simulink model "passiveBalancing"  (R2020b)
settings: Solver=ode23t  StartTime=0.0  StopTime=3600 * 15  MaxStep=.5  RelTol=1e-3  AbsTol=1e-3  EnableMultiTasking=on
PreLoadFcn:
  | passiveBalancing_ini;
model workspace (MAT data in the model file):
  Switch = 1
values from neighbouring files (symbols this model uses):
  I_cc = 4    [passiveBalancing_ini.m]
  I_gain = 10    [passiveBalancing_ini.m]
  P_gain = 100    [passiveBalancing_ini.m]
  R_bleed = 20    [passiveBalancing_ini.m]
  T_f = 600    [passiveBalancing_ini.m]
  V_top = 4.1    [passiveBalancing_ini.m]
libraries: fl_lib x15, nesl_utility x15, ee_lib x6, simulink x1, pid_lib x1
(part 1 of 2)
settings Model: PacingRate=100000  Creator=Amrathesh  LastModifiedBy=amrat
settings SolverCC: AutoScaleAbsTol=off  ZeroCrossAlgorithm=Adaptive
settings DataIOCC: LimitDataPoints=on  SaveOutput=off  SignalLogging=off  SaveTime=off  ReturnWorkspaceOutputs=off
settings OptimizationCC: DefaultParameterBehavior=Inlined  LifeSpan=2  EfficientTunableParamExpr=on
settings DebuggingCC: AlgebraicLoopMsg=error  AllowSymbolicDim=off  PregeneratedLibrarySubsystemCodeDiagnostic=none  SFUnexpectedBacktrackingDiag=warning  SFNoUnconditionalDefaultTransitionDiag=none  SFExecutionAtInitializationDiag=none  ArithmeticOperatorsInVariantConditions=warning
settings HardwareCC: ProdWordSize=32
settings ModelReferenceCC: PropagateSignalLabelsOutOfModel=off
settings SFSimCC: SimUseLocalCustomCode=off  MATLABDynamicMemAlloc=off  CustomCodeUndefinedFunction=UseInterfaceOnly
settings RTWCC: Description=Embedded Coder  SystemTargetFile=ert.tlc  TemplateMakefile=ert_default_tmf  GenerateReport=on  RTWUseLocalCustomCode=off  IncludeHyperlinkInReport=on  LaunchReport=on  GenerateTraceInfo=on  GenerateTraceReport=on  GenerateTraceReportSl=on  GenerateTraceReportSf=on  GenerateTraceReportEml=on
settings CodeAppCC: ForceParamTrailComments=on  IgnoreCustomStorageClasses=off  OperatorAnnotations=on  SimulinkDataObjDesc=on  SFDataObjDesc=on  MATLABFcnDesc=on  InsertBlockDesc=on  StateflowObjectComments=on  MATLABSourceComments=on
settings ERTTargetCC: MultiwordLength=2048  GenerateSampleERTMain=on  InlinedParameterPlacement=NonHierarchical  ERTCustomFileTemplate=example_file_process.tlc
settings ConfigComp: CovMetricSettings=dw  CovSaveCumulativeToWorkspaceVar=on  CovSaveSingleToWorkspaceVar=on  CovExternalEMLEnable=off
settings SimscapeCC: SimscapeNormalizeSystem=off  SimscapeLogType=all  SimscapeLogToSDI=on  SimscapeLogDataHistory=10000

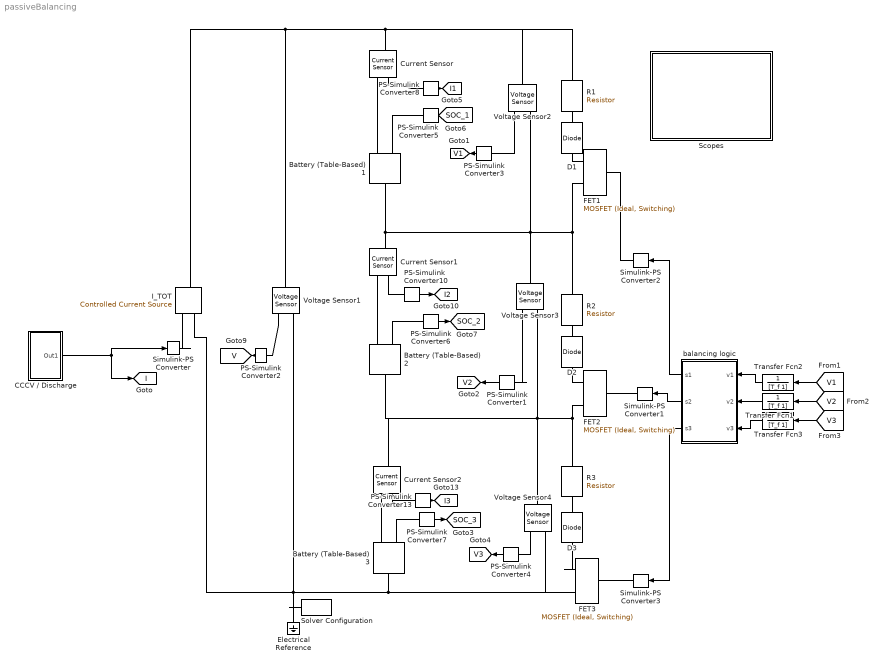
== system passiveBalancing ==
  Battery (Table-Based)1 : ee_lib/Sources/Battery (Table-Based)  Tag={'toolbox/physmod/elec/library/m/ee_lib_parts';'Sources/Battery__Table_Based_/Panasonic/UR18650A.xml'}  SOC_vec=[0.100000000000000;0.200000000000000;0.300000000000000;0.400000000000000;0.500000000000000;0.600000000000000;0.700000000000000;0.800000000000000;0.900000000000000;1]  T_dependence=ee.enum.temperature_dependence.yes  prm_dir=ee.enum.battery.prm_dir.noCurrentDirectionality  T_vec=[278.150000000000,293.150000000000,313.150000000000] K  V0_mat=[3.48407194875853,3.49373906253632,3.50592874552606;3.55418080716149,3.55259570558520,3.55508312112845;3.60440404431230,3.61410230902054,3.61515360383738;3.64321489304947,3.64896659680084,3.65685703896214;3.68502177847119,3.68864192779988,3.69639679484736;3.74422605890089,3.74398921633946,3.75105784288072;3.82967867350671,3.83940080415011,3.85325138336218;3.94315917033962,3.94854312702762,3.95608335309560;4.05943812577673,4.06094828281537,4.06565632904983;4.19049029477082,4.19030181290971,4.18799231154579] V  V0_vec=[2.81006584508995 3.22022478679487 3.35333985530666 3.4210479419583 3.43340289744142 3.44901435079157 3.46164239061189 3.47280320112771 3.47971224601289 3.48236456069527 3.48683507881654 3.49335561249342 3.49763390170867 3.50163709058121 3.50680001394047 3.51219805506247 3.51751682512439 3.52259342518673 3.52865552184197 3.53316807350089 3.53768062515982 3.54219317681874 3.54670572847766 3.55143972547218 3.55647692760588 3.56168247719111 3.56694531744751 3.57220815770393 3.57747099796033 3.58273383821674 3.5875530992875 3.59176313859395 3.59524803726717 3.59891401218516 3.60257998710315 3.60624596202113 3.61006223866338 3.61403025053352 3.61799826240367 3.62196627427381 3.62727855718798 3.6319884367608 3.63698876786423 3.64203407138805 3.64707937491187 3.65212467843569 3.65716998195951 3.66221528548332 3.66729939294707 3.67295160796092 3.67881814753232 3.68468468710373 3.69055122667513 3.69641776624653 3.70184846811763 3.70677938326847 3.71171029841932 3.71666876915231 3.72316392974375 3.7304733189824 3.73778270822105 3.745036871918 3.75209516011368 3.75915344830935 3.76621173650503 3.77398066542743 3.78333553443086 3.7926451126744 3.80054605529622 3.80844699791802 3.81634794053984 3.82429836269964 3.83446027504896 3.84531418436014 3.85639886265616 3.86778116509702 3.87916346753789 3.89054576997875 3.90044812182432 3.91099190865954 3.92153569549475 3.93213383878664 3.94271770825583 3.95339662764836 3.96407554704089 3.97475446643342 3.9856014296663 3.99763743545176 4.00976952670118 4.02190161795059 4.03372971668446 4.04698942952056 4.06070820502709 4.07426940349866 4.08362358507044 4.0946516607131 4.10632109738002 4.11746763572909 4.13600949794925 4.11358192572688] V  R0_mat=[0.0164025520353838,0.00991391593917779,0.00933168437168862;0.0119600956597842,0.00875043635238341,0.00956154423893035;0.0119853068610826,0.00832297953681552,0.00854455182155223;0.0111330643324705,0.00872061850253288,0.00956139374993682;0.0118222895857250,0.00795909444960185,0.00880754790179610;0.0116748342939053,0.00856548056926203,0.00938193010301517;0.0112768580015193,0.00843330788647423,0.00996649091964517;0.0118933795996695,0.00850334186162495,0.00960019659194077;0.0120321348242062,0.00846602435735512,0.00963753251603531;0.0124098156482057,0.00846539753229566,0.00929821710866923] Ohm  R0_vec=[0.056515741669998 0.0979844967251839 0.0915569898783186 0.0798231515434287 0.0702524951827934 0.0654000373090211 0.063093856936673 0.0616308263389111 0.0599710561216984 0.057768198464152 0.0561995978201733 0.0555761442485201 0.0546523884163435 0.0536806499662514 0.0531134700580429 0.0526283079740431 0.0521431458900432 0.0516579838060416 0.0515369348195236 0.0512705771965729 0.0510042195736231 0.0507378619506724 0.0504715043277217 0.0502823950776516 0.0502561644624615 0.0502595683975375 0.0502729648915397 0.0502863613855435 0.0502997578795457 0.0503131543735487 0.0503265508675508 0.0502574673059781 0.0501120429454529 0.0500297847168234 0.0499475264881939 0.0498652682595635 0.0497830100309331 0.0497007518023036 0.0496184935736741 0.0495362353450446 0.0496803807796349 0.0495816760338741 0.0494829712881124 0.0493842665423516 0.0492855617965899 0.04918685705083 0.0490881523050684 0.0489894475593067 0.0488907428135468 0.0488792431935741 0.0489051257638717 0.0489310083341703 0.0489568909044689 0.0489827734747674 0.048856619637978 0.0485561215964543 0.0482556235549287 0.0479551255134041 0.0478887983616394 0.047964487834391 0.0480401773071417 0.0480966020560407 0.0480846981417065 0.0480727942273722 0.048060890313038 0.0481036878566563 0.04837530229414 0.0486311176293377 0.0483955484453293 0.0481599792613174 0.0479244100773082 0.0476974710452733 0.0478971482990236 0.0483382198417974 0.0487792913845713 0.0492203629273451 0.0496614344701189 0.0501025060128928 0.0499772096727922 0.0499177661458976 0.049858322619003 0.0497988790921067 0.0497828516280938 0.0498086176006431 0.0498343835731925 0.0498601495457418 0.0499152254904454 0.0500578808408836 0.0502005361913236 0.0503431915417627 0.0503798029914302 0.0505673178409918 0.0508126169361116 0.0509278793074452 0.049575577643969 0.0485152342486694 0.0475667561482966 0.0457576853133315 0.0447350638775861 0.0121745905370672] Ohm  R0_dis_mat=[0.03 0.015 0.002;0.04 0.017 0.008;0.039 0.012 0.006;0.027 0.013 0.021] % Parameter not set Ohm  R0_dis_vec=[0.015 0.017 0.012 0.013] % Parameter not set Ohm  R0_ch_mat=[0.03 0.015 0.002;0.04 0.017 0.008;0.039 0.012 0.006;0.027 0.013 0.021] % Parameter not set Ohm  R0_ch_vec=[0.015 0.017 0.012 0.013] % Parameter not set Ohm  AH_vec=[1.82394991873531 2.0165 2.32772554803559] hr*A  AH=2.05260817612401 hr*A  prm_leak=ee.enum.battery.prm_leak.disabled  Rleak_vec=[8000 7000 6000] % Parameter not set Ohm  Rleak=7000 % Parameter not set Ohm  extrapolation_option=ee.enum.extrapolation.linear  prm_dyn=ee.enum.battery.prm_dyn.rc3  R1_mat=[0.00470517937000299,0.000293638394729167,0.000948546678306262;0.00290275050725254,0.000906415294998030,0.000287127543931831;0.00173884757466172,0.00126508138885500,0.00118355047696410;0.00166867739185738,0.000314621823867429,0.000269194023197089;0.000922417169458259,0.00115254740207724,0.000615957962246520;0.00120601315196432,0.000484496431848577,0.000263719105084760;0.00134107014418335,0.000722662778209487,4.84440937939109e-05;0.00102728323615524,0.000788593565891369,0.000287482375984320;0.00107112644740310,0.000808964645885711,0.000207425991333054;0.00109762911159868,0.000794632163172680,0.000106864004690497] Ohm  R1_vec=[0.076 0.022 0.007 0.043] % Parameter not set Ohm  tau1_mat=[13.5871605581300,9.71544043458337,4.31542721208131;12.5481735435305,12.1200192117783,22.7640233955017;7.48337010487386,12.0370710856561,8.29042934523224;9.44542449719648,10.9054745144726,9.51113592097300;9.24780665009956,9.25131458132309,4.68694878468948;13.0193706450093,13.4646058128269,7.73065506391290;11.2694049052077,10.2523357120003,10.8430353394808;10.5849479160592,10.0421839086956,10.9678971839482;9.25375749656255,9.65077226703459,11.6975516144793;10.0189550950196,10.0848834113777,9.87774425333310] s  tau1_vec=[148 110 27 22] % Parameter not set s  R2_mat=[0.000684064694305059,0.000979420886572540,0.000510171787438108;0.00251991269966880,0.000998429425096649,0.000143514073100964;0.00146068562126075,0.00101421826179247,0.000570655533199722;0.00169830619514015,0.00108683386499324,0.000208423134005952;0.00167031143922319,0.000980618529905995,0.000651263003556613;0.000940978707058922,0.000878005470765354,0.000327115321338108;0.000987171552806869,0.000893842003198636,9.25394354022508e-05;0.00105023394930685,0.000992613735542309,0.000107350277866256;0.00104040490708932,0.000868081363505911,9.60282071092013e-05;0.000906032230510198,0.000913369768442737,0.000476753719169488] Ohm  R2_vec=[0.382 0.006 0.007 0.956] % Parameter not set Ohm  tau2_mat=[50.0886429204366,61.4453898981661,145.884876037851;74.6890198323087,50.4659345461731,86.1376304381821;97.3437456249129,84.5850607625997,46.7659950347051;69.5883917264204,54.8647909590588,95.8259882470036;84.2274457727954,55.6603698124908,49.8887181712856;85.6679398764468,66.7955372911173,100.658737711864;91.0542017364846,92.0037411543702,98.7286168651434;105.401951521745,81.0404007236597,142.459568124630;96.5977974872106,90.8335209230926,115.401022170525;93.3993331962355,104.582879809587,83.7886054703847] s  tau2_vec=[44 24 14 13419] % Parameter not set s  R3_mat=[0.00647728107284730,0.00265301875816448,0.00382437341121983;0.00361737977004768,0.00111981676039765,0.00335084458017034;0.00344585619669106,0.00161752813625906,6.99540921903032e-05;0.00315346597824661,0.00130153280759591,0.00128660807490130;0.00209410692411210,0.00175471389437080,0.000316666511381357;0.00191509386455154,0.000370366587789619,0.000335793536625847;0.000572834619148222,0.000925138687019395,0.000330091526981303;0.00113886835462710,0.000867792101494099,0.000801284291305556;0.00101072488301601,0.000662353437832612,1.76827486513599e-05;0.00109338554767636,0.000329888238858683,7.93589066577793e-05] Ohm  R3_vec=[0.382 0.006 0.007 0.956] % Parameter not set Ohm  tau3_mat=[701.994643225609,650.007334256828,4085.79825438844;925.823429071832,649.854940905500,4973.41475833222;789.333229923387,938.725273795671,279.002198521502;654.594564127694,349.419044951255,894.440824445244;541.309382097595,983.444269794273,2138.18581380245;689.289031846017,958.570032564448,882.678111947643;601.673035616931,962.088556655044,358.867760831677;466.377911573388,402.220930598748,253.373956799259;329.012511634609,405.712600993442,527.026256725996;499.960911848800,568.259886582724,628.422969338960] s  tau3_vec=[44 24 14 13419] % Parameter not set s  R4_mat=[0.014 0.382 0.407;0.028 0.006 0.007;0.014 0.007 0.006;0.333 0.956 0.912] % Parameter not set Ohm  R4_vec=[0.382 0.006 0.007 0.956] % Parameter not set Ohm  tau4_mat=[1 44 5644;11 24 506;2 14 330;3310 13419 30216] % Parameter not set s  tau4_vec=[44 24 14 13419] % Parameter not set s  R5_mat=[0.014 0.382 0.407;0.028 0.006 0.007;0.014 0.007 0.006;0.333 0.956 0.912] % Parameter not set Ohm  R5_vec=[0.382 0.006 0.007 0.956] % Parameter not set Ohm  tau5_mat=[1 44 5644;11 24 506;2 14 330;3310 13419 30216] % Parameter not set s  tau5_vec=[44 24 14 13419] % Parameter not set s  prm_fade=ee.enum.battery.prm_fade.equations  N0=100 % Parameter not set  dV0=0 % Parameter not set  dR0=0 % Parameter not set  dAH=0 % Parameter not set  dRleak=0 % Parameter not set  dR1=0 % Parameter not set  dR2=0 % Parameter not set  dR3=0 % Parameter not set  dR4=0 % Parameter not set  dR5=0 % Parameter not set  N0vec=[1 7 13 19 25 31 37 43 49 55 61 67 73 79 85 91 97 103 109 115 121 127 133 139 145 151 157 163 169 175 181 187 193 199 205 211 217 223 229 235 241 247 253 259 265 271 277 283 289 295 301 307 313 319 325 331 337 343 349 355 361 367 373 379 385 391 397 403 409 415 421 427 433 439 445 451 457 463 469 475 481 487 493 499]  Tfadevec=[298.15 323.15] % Parameter not set K  dV0vec=[0 0.11971976024812 0.239439520496219 0.359159280744318 0.478879040992438 0.501067226691431 0.402089625480699 0.303112024269989 0.204134423059257 0.107430319615636 0.0613178904713528 0.0203784059293676 -0.0205610786126608 -0.061500563154646 -0.102440047696653 -0.14337953223866 -0.201539559021902 -0.314370645177291 -0.4272017313327 -0.535644559188378 -0.642274363906691 -0.745773535175882 -0.83621855809896 -0.926663581022039 -1.04473766830393 -1.17586008635983 -1.2842177466678 -1.38421479409414 -1.48422494017385 -1.58423508625356 -1.68205677034908 -1.77872034043833 -1.87538391052757 -1.96871527598932 -2.05494235082241 -2.14116942565553 -2.22342333172441 -2.30746775676303 -2.3916483637309 -2.47582897069879 -2.56000957766668 -2.64419018463457 -2.72837079160248 -2.81255139857038 -2.89611302552253 -2.97962692693163 -3.06874730213896 -3.15533627389878 -3.23773436162621 -3.32013244935364 -3.4021017936101 -3.48322334975892 -3.56434490590772 -3.64546646205654 -3.72658801820533 -3.8077095743541 -3.86254494056368 -3.91405004441099 -3.96555514825832 -4.01706025210565 -4.06856535595298 -4.1200704598003 -4.17141610474255 -4.23129042669511 -4.30051147066416 -4.36973251463322 -4.43899132382803 -4.50830572201986 -4.57762012021168 -4.64693451840349 -4.7160044748888 -4.7804348165123 -4.8441936541821 -4.9079524918519 -4.97171132952168 -5.03547016719147 -5.09922900486127 -5.16844365985214 -5.2420874206298 -5.31495381814591 -5.38782021566204 -5.46647669730484 -5.55023330252746 -5.63398990775009]  dR0vec=[0;0;0;0;0;0;0;0;0;0;0;0;0;0;0;0;0;0;0;0;0;0;0;0;0;0;0;0;0;0;0;0;0;0;0;0;0;0;0;0;0;0;0;0;0;0;0;0;0;0;0;0;0;0;0;0;0;0;0;0;0;0;0;0;0;0;0;0;0;0;0;0;0;0;0;0;0;0;0;0;0;0;0;0] % Parameter not set  dAHvec=[0 -0.219585533835757 -0.439171067671514 -0.658756601507271 -0.878342135343028 -1.09792766917876 -1.31751320301452 -1.53709873685028 -1.75668427068601 -1.97122596415023 -2.1223113669781 -2.27339676980596 -2.42448217263385 -2.57556757546173 -2.7266529782896 -2.87773838111746 -3.08823618102998 -3.48597596052145 -3.88371574001296 -4.28145551950445 -4.67919529899595 -5.07693507848744 -5.47467485797895 -5.87241463747045 -6.27015441696194 -6.66789419645344 -6.9965805687467 -7.29646150863608 -7.59634244852543 -7.89622338841479 -8.19610432830414 -8.49598526819352 -8.79586620808287 -9.09574714797224 -9.3956280878616 -9.69550902775097 -9.98157206200379 -10.2670000366216 -10.5524280112395 -10.8378559858573 -11.1232839604752 -11.408711935093 -11.6941399097109 -11.9795678843287 -12.2649958589466 -12.5504238335644 -12.8550132224376 -13.1674981798519 -13.4799831372661 -13.7924680946804 -14.1049530520947 -14.417438009509 -14.7299229669232 -15.0424079243375 -15.3548928817518 -15.6673778391661 -15.8786068624772 -16.0770075212716 -16.275408180066 -16.4738088388604 -16.6722094976548 -16.8706101564492 -17.0690108152436 -17.3017214786887 -17.5707595995574 -17.8397977204261 -18.1088358412948 -18.3778739621634 -18.6469120830321 -18.9159502039008 -19.1849883247695 -19.4363586274065 -19.6851091060939 -19.9338595847813 -20.1826100634686 -20.431360542156 -20.6801110208434 -20.9501469749229 -21.252844657746 -21.5555423405691 -21.8582400233922 -22.1609377062153 -22.4636353890384 -22.7663330718615]  dRleakvec=[0 0 0] % Parameter not set  dR1vec=[0 0 0] % Parameter not set  dR2vec=[0 0 0] % Parameter not set  dR3vec=[0 0 0] % Parameter not set  dR4vec=[0 0 0] % Parameter not set  dR5vec=[0 0 0] % Parameter not set  dV0mat=[0 0;0 0;0 0] % Parameter not set  dR0mat=[0 0;0 0;0 0] % Parameter not set  dAHmat=[0 0;0 0;0 0] % Parameter not set  dRleakmat=[0 0;0 0;0 0] % Parameter not set  dR1mat=[0 0;0 0;0 0] % Parameter not set  dR2mat=[0 0;0 0;0 0] % Parameter not set  dR3mat=[0 0;0 0;0 0] % Parameter not set  dR4mat=[0 0;0 0;0 0] % Parameter not set  dR5mat=[0 0;0 0;0 0] % Parameter not set  temperature=298.15 K  i_specify=off  i_priority=None  i=0 A  i_nominal_specify=off  i_nominal_unit=A  i_nominal_value=1  v_specify=off  v_priority=None  v=0 V  v_nominal_specify=off  v_nominal_unit=V  v_nominal_value=1  stateOfCharge_specify=on  stateOfCharge_priority=High  stateOfCharge=0.8  stateOfCharge_nominal_specify=off  stateOfCharge_nominal_unit=1  stateOfCharge_nominal_value=1  num_cycles_specify=off  num_cycles_priority=High  num_cycles=0  num_cycles_nominal_specify=off  num_cycles_nominal_unit=1  num_cycles_nominal_value=1  thermal_mass=30000 J/K  temperature_specify=off  temperature_priority=High  temperature_nominal_specify=off  temperature_nominal_unit=K  temperature_nominal_value=1
      settings: AttributesFormatString=UR18650A  SourceProductBaseCode=PS  InternalSimscapePortConfiguration="{\"Bottom\":[],\"Left\":[{\"id\":\"p\",\"label\":\"+\",\"type\":\"foundation.electrical.electrical\"},{\"id\":\"soc\",\"label\":\"SOC\",\"type\":\"output\"}],\"Right\":[{\"id\":\"n\",\"label\":\"-\",\"type\":\"foundation.electrical.electrical\"}],\"Top\":[]}"
  Battery (Table-Based)2 : ee_lib/Sources/Battery (Table-Based)  Tag={'toolbox/physmod/elec/library/m/ee_lib_parts';'Sources/Battery__Table_Based_/Panasonic/UR18650A.xml'}  SOC_vec=[0.100000000000000;0.200000000000000;0.300000000000000;0.400000000000000;0.500000000000000;0.600000000000000;0.700000000000000;0.800000000000000;0.900000000000000;1]  T_dependence=ee.enum.temperature_dependence.yes  prm_dir=ee.enum.battery.prm_dir.noCurrentDirectionality  T_vec=[278.150000000000,293.150000000000,313.150000000000] K  V0_mat=[3.48407194875853,3.49373906253632,3.50592874552606;3.55418080716149,3.55259570558520,3.55508312112845;3.60440404431230,3.61410230902054,3.61515360383738;3.64321489304947,3.64896659680084,3.65685703896214;3.68502177847119,3.68864192779988,3.69639679484736;3.74422605890089,3.74398921633946,3.75105784288072;3.82967867350671,3.83940080415011,3.85325138336218;3.94315917033962,3.94854312702762,3.95608335309560;4.05943812577673,4.06094828281537,4.06565632904983;4.19049029477082,4.19030181290971,4.18799231154579] V  V0_vec=[2.81006584508995 3.22022478679487 3.35333985530666 3.4210479419583 3.43340289744142 3.44901435079157 3.46164239061189 3.47280320112771 3.47971224601289 3.48236456069527 3.48683507881654 3.49335561249342 3.49763390170867 3.50163709058121 3.50680001394047 3.51219805506247 3.51751682512439 3.52259342518673 3.52865552184197 3.53316807350089 3.53768062515982 3.54219317681874 3.54670572847766 3.55143972547218 3.55647692760588 3.56168247719111 3.56694531744751 3.57220815770393 3.57747099796033 3.58273383821674 3.5875530992875 3.59176313859395 3.59524803726717 3.59891401218516 3.60257998710315 3.60624596202113 3.61006223866338 3.61403025053352 3.61799826240367 3.62196627427381 3.62727855718798 3.6319884367608 3.63698876786423 3.64203407138805 3.64707937491187 3.65212467843569 3.65716998195951 3.66221528548332 3.66729939294707 3.67295160796092 3.67881814753232 3.68468468710373 3.69055122667513 3.69641776624653 3.70184846811763 3.70677938326847 3.71171029841932 3.71666876915231 3.72316392974375 3.7304733189824 3.73778270822105 3.745036871918 3.75209516011368 3.75915344830935 3.76621173650503 3.77398066542743 3.78333553443086 3.7926451126744 3.80054605529622 3.80844699791802 3.81634794053984 3.82429836269964 3.83446027504896 3.84531418436014 3.85639886265616 3.86778116509702 3.87916346753789 3.89054576997875 3.90044812182432 3.91099190865954 3.92153569549475 3.93213383878664 3.94271770825583 3.95339662764836 3.96407554704089 3.97475446643342 3.9856014296663 3.99763743545176 4.00976952670118 4.02190161795059 4.03372971668446 4.04698942952056 4.06070820502709 4.07426940349866 4.08362358507044 4.0946516607131 4.10632109738002 4.11746763572909 4.13600949794925 4.11358192572688] V  R0_mat=[0.0164025520353838,0.00991391593917779,0.00933168437168862;0.0119600956597842,0.00875043635238341,0.00956154423893035;0.0119853068610826,0.00832297953681552,0.00854455182155223;0.0111330643324705,0.00872061850253288,0.00956139374993682;0.0118222895857250,0.00795909444960185,0.00880754790179610;0.0116748342939053,0.00856548056926203,0.00938193010301517;0.0112768580015193,0.00843330788647423,0.00996649091964517;0.0118933795996695,0.00850334186162495,0.00960019659194077;0.0120321348242062,0.00846602435735512,0.00963753251603531;0.0124098156482057,0.00846539753229566,0.00929821710866923] Ohm  R0_vec=[0.056515741669998 0.0979844967251839 0.0915569898783186 0.0798231515434287 0.0702524951827934 0.0654000373090211 0.063093856936673 0.0616308263389111 0.0599710561216984 0.057768198464152 0.0561995978201733 0.0555761442485201 0.0546523884163435 0.0536806499662514 0.0531134700580429 0.0526283079740431 0.0521431458900432 0.0516579838060416 0.0515369348195236 0.0512705771965729 0.0510042195736231 0.0507378619506724 0.0504715043277217 0.0502823950776516 0.0502561644624615 0.0502595683975375 0.0502729648915397 0.0502863613855435 0.0502997578795457 0.0503131543735487 0.0503265508675508 0.0502574673059781 0.0501120429454529 0.0500297847168234 0.0499475264881939 0.0498652682595635 0.0497830100309331 0.0497007518023036 0.0496184935736741 0.0495362353450446 0.0496803807796349 0.0495816760338741 0.0494829712881124 0.0493842665423516 0.0492855617965899 0.04918685705083 0.0490881523050684 0.0489894475593067 0.0488907428135468 0.0488792431935741 0.0489051257638717 0.0489310083341703 0.0489568909044689 0.0489827734747674 0.048856619637978 0.0485561215964543 0.0482556235549287 0.0479551255134041 0.0478887983616394 0.047964487834391 0.0480401773071417 0.0480966020560407 0.0480846981417065 0.0480727942273722 0.048060890313038 0.0481036878566563 0.04837530229414 0.0486311176293377 0.0483955484453293 0.0481599792613174 0.0479244100773082 0.0476974710452733 0.0478971482990236 0.0483382198417974 0.0487792913845713 0.0492203629273451 0.0496614344701189 0.0501025060128928 0.0499772096727922 0.0499177661458976 0.049858322619003 0.0497988790921067 0.0497828516280938 0.0498086176006431 0.0498343835731925 0.0498601495457418 0.0499152254904454 0.0500578808408836 0.0502005361913236 0.0503431915417627 0.0503798029914302 0.0505673178409918 0.0508126169361116 0.0509278793074452 0.049575577643969 0.0485152342486694 0.0475667561482966 0.0457576853133315 0.0447350638775861 0.0121745905370672] Ohm  R0_dis_mat=[0.03 0.015 0.002;0.04 0.017 0.008;0.039 0.012 0.006;0.027 0.013 0.021] % Parameter not set Ohm  R0_dis_vec=[0.015 0.017 0.012 0.013] % Parameter not set Ohm  R0_ch_mat=[0.03 0.015 0.002;0.04 0.017 0.008;0.039 0.012 0.006;0.027 0.013 0.021] % Parameter not set Ohm  R0_ch_vec=[0.015 0.017 0.012 0.013] % Parameter not set Ohm  AH_vec=[1.82394991873531 2.0165 2.32772554803559] hr*A  AH=2.05260817612401 hr*A  prm_leak=ee.enum.battery.prm_leak.disabled  Rleak_vec=[8000 7000 6000] % Parameter not set Ohm  Rleak=7000 % Parameter not set Ohm  extrapolation_option=ee.enum.extrapolation.linear  prm_dyn=ee.enum.battery.prm_dyn.rc3  R1_mat=[0.00470517937000299,0.000293638394729167,0.000948546678306262;0.00290275050725254,0.000906415294998030,0.000287127543931831;0.00173884757466172,0.00126508138885500,0.00118355047696410;0.00166867739185738,0.000314621823867429,0.000269194023197089;0.000922417169458259,0.00115254740207724,0.000615957962246520;0.00120601315196432,0.000484496431848577,0.000263719105084760;0.00134107014418335,0.000722662778209487,4.84440937939109e-05;0.00102728323615524,0.000788593565891369,0.000287482375984320;0.00107112644740310,0.000808964645885711,0.000207425991333054;0.00109762911159868,0.000794632163172680,0.000106864004690497] Ohm  R1_vec=[0.076 0.022 0.007 0.043] % Parameter not set Ohm  tau1_mat=[13.5871605581300,9.71544043458337,4.31542721208131;12.5481735435305,12.1200192117783,22.7640233955017;7.48337010487386,12.0370710856561,8.29042934523224;9.44542449719648,10.9054745144726,9.51113592097300;9.24780665009956,9.25131458132309,4.68694878468948;13.0193706450093,13.4646058128269,7.73065506391290;11.2694049052077,10.2523357120003,10.8430353394808;10.5849479160592,10.0421839086956,10.9678971839482;9.25375749656255,9.65077226703459,11.6975516144793;10.0189550950196,10.0848834113777,9.87774425333310] s  tau1_vec=[148 110 27 22] % Parameter not set s  R2_mat=[0.000684064694305059,0.000979420886572540,0.000510171787438108;0.00251991269966880,0.000998429425096649,0.000143514073100964;0.00146068562126075,0.00101421826179247,0.000570655533199722;0.00169830619514015,0.00108683386499324,0.000208423134005952;0.00167031143922319,0.000980618529905995,0.000651263003556613;0.000940978707058922,0.000878005470765354,0.000327115321338108;0.000987171552806869,0.000893842003198636,9.25394354022508e-05;0.00105023394930685,0.000992613735542309,0.000107350277866256;0.00104040490708932,0.000868081363505911,9.60282071092013e-05;0.000906032230510198,0.000913369768442737,0.000476753719169488] Ohm  R2_vec=[0.382 0.006 0.007 0.956] % Parameter not set Ohm  tau2_mat=[50.0886429204366,61.4453898981661,145.884876037851;74.6890198323087,50.4659345461731,86.1376304381821;97.3437456249129,84.5850607625997,46.7659950347051;69.5883917264204,54.8647909590588,95.8259882470036;84.2274457727954,55.6603698124908,49.8887181712856;85.6679398764468,66.7955372911173,100.658737711864;91.0542017364846,92.0037411543702,98.7286168651434;105.401951521745,81.0404007236597,142.459568124630;96.5977974872106,90.8335209230926,115.401022170525;93.3993331962355,104.582879809587,83.7886054703847] s  tau2_vec=[44 24 14 13419] % Parameter not set s  R3_mat=[0.00647728107284730,0.00265301875816448,0.00382437341121983;0.00361737977004768,0.00111981676039765,0.00335084458017034;0.00344585619669106,0.00161752813625906,6.99540921903032e-05;0.00315346597824661,0.00130153280759591,0.00128660807490130;0.00209410692411210,0.00175471389437080,0.000316666511381357;0.00191509386455154,0.000370366587789619,0.000335793536625847;0.000572834619148222,0.000925138687019395,0.000330091526981303;0.00113886835462710,0.000867792101494099,0.000801284291305556;0.00101072488301601,0.000662353437832612,1.76827486513599e-05;0.00109338554767636,0.000329888238858683,7.93589066577793e-05] Ohm  R3_vec=[0.382 0.006 0.007 0.956] % Parameter not set Ohm  tau3_mat=[701.994643225609,650.007334256828,4085.79825438844;925.823429071832,649.854940905500,4973.41475833222;789.333229923387,938.725273795671,279.002198521502;654.594564127694,349.419044951255,894.440824445244;541.309382097595,983.444269794273,2138.18581380245;689.289031846017,958.570032564448,882.678111947643;601.673035616931,962.088556655044,358.867760831677;466.377911573388,402.220930598748,253.373956799259;329.012511634609,405.712600993442,527.026256725996;499.960911848800,568.259886582724,628.422969338960] s  tau3_vec=[44 24 14 13419] % Parameter not set s  R4_mat=[0.014 0.382 0.407;0.028 0.006 0.007;0.014 0.007 0.006;0.333 0.956 0.912] % Parameter not set Ohm  R4_vec=[0.382 0.006 0.007 0.956] % Parameter not set Ohm  tau4_mat=[1 44 5644;11 24 506;2 14 330;3310 13419 30216] % Parameter not set s  tau4_vec=[44 24 14 13419] % Parameter not set s  R5_mat=[0.014 0.382 0.407;0.028 0.006 0.007;0.014 0.007 0.006;0.333 0.956 0.912] % Parameter not set Ohm  R5_vec=[0.382 0.006 0.007 0.956] % Parameter not set Ohm  tau5_mat=[1 44 5644;11 24 506;2 14 330;3310 13419 30216] % Parameter not set s  tau5_vec=[44 24 14 13419] % Parameter not set s  prm_fade=ee.enum.battery.prm_fade.equations  N0=100 % Parameter not set  dV0=0 % Parameter not set  dR0=0 % Parameter not set  dAH=0 % Parameter not set  dRleak=0 % Parameter not set  dR1=0 % Parameter not set  dR2=0 % Parameter not set  dR3=0 % Parameter not set  dR4=0 % Parameter not set  dR5=0 % Parameter not set  N0vec=[1 7 13 19 25 31 37 43 49 55 61 67 73 79 85 91 97 103 109 115 121 127 133 139 145 151 157 163 169 175 181 187 193 199 205 211 217 223 229 235 241 247 253 259 265 271 277 283 289 295 301 307 313 319 325 331 337 343 349 355 361 367 373 379 385 391 397 403 409 415 421 427 433 439 445 451 457 463 469 475 481 487 493 499]  Tfadevec=[298.15 323.15] % Parameter not set K  dV0vec=[0 0.11971976024812 0.239439520496219 0.359159280744318 0.478879040992438 0.501067226691431 0.402089625480699 0.303112024269989 0.204134423059257 0.107430319615636 0.0613178904713528 0.0203784059293676 -0.0205610786126608 -0.061500563154646 -0.102440047696653 -0.14337953223866 -0.201539559021902 -0.314370645177291 -0.4272017313327 -0.535644559188378 -0.642274363906691 -0.745773535175882 -0.83621855809896 -0.926663581022039 -1.04473766830393 -1.17586008635983 -1.2842177466678 -1.38421479409414 -1.48422494017385 -1.58423508625356 -1.68205677034908 -1.77872034043833 -1.87538391052757 -1.96871527598932 -2.05494235082241 -2.14116942565553 -2.22342333172441 -2.30746775676303 -2.3916483637309 -2.47582897069879 -2.56000957766668 -2.64419018463457 -2.72837079160248 -2.81255139857038 -2.89611302552253 -2.97962692693163 -3.06874730213896 -3.15533627389878 -3.23773436162621 -3.32013244935364 -3.4021017936101 -3.48322334975892 -3.56434490590772 -3.64546646205654 -3.72658801820533 -3.8077095743541 -3.86254494056368 -3.91405004441099 -3.96555514825832 -4.01706025210565 -4.06856535595298 -4.1200704598003 -4.17141610474255 -4.23129042669511 -4.30051147066416 -4.36973251463322 -4.43899132382803 -4.50830572201986 -4.57762012021168 -4.64693451840349 -4.7160044748888 -4.7804348165123 -4.8441936541821 -4.9079524918519 -4.97171132952168 -5.03547016719147 -5.09922900486127 -5.16844365985214 -5.2420874206298 -5.31495381814591 -5.38782021566204 -5.46647669730484 -5.55023330252746 -5.63398990775009]  dR0vec=[0;0;0;0;0;0;0;0;0;0;0;0;0;0;0;0;0;0;0;0;0;0;0;0;0;0;0;0;0;0;0;0;0;0;0;0;0;0;0;0;0;0;0;0;0;0;0;0;0;0;0;0;0;0;0;0;0;0;0;0;0;0;0;0;0;0;0;0;0;0;0;0;0;0;0;0;0;0;0;0;0;0;0;0] % Parameter not set  dAHvec=[0 -0.219585533835757 -0.439171067671514 -0.658756601507271 -0.878342135343028 -1.09792766917876 -1.31751320301452 -1.53709873685028 -1.75668427068601 -1.97122596415023 -2.1223113669781 -2.27339676980596 -2.42448217263385 -2.57556757546173 -2.7266529782896 -2.87773838111746 -3.08823618102998 -3.48597596052145 -3.88371574001296 -4.28145551950445 -4.67919529899595 -5.07693507848744 -5.47467485797895 -5.87241463747045 -6.27015441696194 -6.66789419645344 -6.9965805687467 -7.29646150863608 -7.59634244852543 -7.89622338841479 -8.19610432830414 -8.49598526819352 -8.79586620808287 -9.09574714797224 -9.3956280878616 -9.69550902775097 -9.98157206200379 -10.2670000366216 -10.5524280112395 -10.8378559858573 -11.1232839604752 -11.408711935093 -11.6941399097109 -11.9795678843287 -12.2649958589466 -12.5504238335644 -12.8550132224376 -13.1674981798519 -13.4799831372661 -13.7924680946804 -14.1049530520947 -14.417438009509 -14.7299229669232 -15.0424079243375 -15.3548928817518 -15.6673778391661 -15.8786068624772 -16.0770075212716 -16.275408180066 -16.4738088388604 -16.6722094976548 -16.8706101564492 -17.0690108152436 -17.3017214786887 -17.5707595995574 -17.8397977204261 -18.1088358412948 -18.3778739621634 -18.6469120830321 -18.9159502039008 -19.1849883247695 -19.4363586274065 -19.6851091060939 -19.9338595847813 -20.1826100634686 -20.431360542156 -20.6801110208434 -20.9501469749229 -21.252844657746 -21.5555423405691 -21.8582400233922 -22.1609377062153 -22.4636353890384 -22.7663330718615]  dRleakvec=[0 0 0] % Parameter not set  dR1vec=[0 0 0] % Parameter not set  dR2vec=[0 0 0] % Parameter not set  dR3vec=[0 0 0] % Parameter not set  dR4vec=[0 0 0] % Parameter not set  dR5vec=[0 0 0] % Parameter not set  dV0mat=[0 0;0 0;0 0] % Parameter not set  dR0mat=[0 0;0 0;0 0] % Parameter not set  dAHmat=[0 0;0 0;0 0] % Parameter not set  dRleakmat=[0 0;0 0;0 0] % Parameter not set  dR1mat=[0 0;0 0;0 0] % Parameter not set  dR2mat=[0 0;0 0;0 0] % Parameter not set  dR3mat=[0 0;0 0;0 0] % Parameter not set  dR4mat=[0 0;0 0;0 0] % Parameter not set  dR5mat=[0 0;0 0;0 0] % Parameter not set  temperature=298.15 K  i_specify=off  i_priority=None  i=0 A  i_nominal_specify=off  i_nominal_unit=A  i_nominal_value=1  v_specify=off  v_priority=None  v=0 V  v_nominal_specify=off  v_nominal_unit=V  v_nominal_value=1  stateOfCharge_specify=on  stateOfCharge_priority=High  stateOfCharge=0.2  stateOfCharge_nominal_specify=off  stateOfCharge_nominal_unit=1  stateOfCharge_nominal_value=1  num_cycles_specify=off  num_cycles_priority=High  num_cycles=0  num_cycles_nominal_specify=off  num_cycles_nominal_unit=1  num_cycles_nominal_value=1  thermal_mass=30000 J/K  temperature_specify=off  temperature_priority=High  temperature_nominal_specify=off  temperature_nominal_unit=K  temperature_nominal_value=1
      settings: AttributesFormatString=UR18650A  SourceProductBaseCode=PS  InternalSimscapePortConfiguration="{\"Bottom\":[],\"Left\":[{\"id\":\"p\",\"label\":\"+\",\"type\":\"foundation.electrical.electrical\"},{\"id\":\"soc\",\"label\":\"SOC\",\"type\":\"output\"}],\"Right\":[{\"id\":\"n\",\"label\":\"-\",\"type\":\"foundation.electrical.electrical\"}],\"Top\":[]}"
  Battery (Table-Based)3 : ee_lib/Sources/Battery (Table-Based)  Tag={'toolbox/physmod/elec/library/m/ee_lib_parts';'Sources/Battery__Table_Based_/Panasonic/UR18650A.xml'}  SOC_vec=[0.100000000000000;0.200000000000000;0.300000000000000;0.400000000000000;0.500000000000000;0.600000000000000;0.700000000000000;0.800000000000000;0.900000000000000;1]  T_dependence=ee.enum.temperature_dependence.yes  prm_dir=ee.enum.battery.prm_dir.noCurrentDirectionality  T_vec=[278.150000000000,293.150000000000,313.150000000000] K  V0_mat=[3.48407194875853,3.49373906253632,3.50592874552606;3.55418080716149,3.55259570558520,3.55508312112845;3.60440404431230,3.61410230902054,3.61515360383738;3.64321489304947,3.64896659680084,3.65685703896214;3.68502177847119,3.68864192779988,3.69639679484736;3.74422605890089,3.74398921633946,3.75105784288072;3.82967867350671,3.83940080415011,3.85325138336218;3.94315917033962,3.94854312702762,3.95608335309560;4.05943812577673,4.06094828281537,4.06565632904983;4.19049029477082,4.19030181290971,4.18799231154579] V  V0_vec=[2.81006584508995 3.22022478679487 3.35333985530666 3.4210479419583 3.43340289744142 3.44901435079157 3.46164239061189 3.47280320112771 3.47971224601289 3.48236456069527 3.48683507881654 3.49335561249342 3.49763390170867 3.50163709058121 3.50680001394047 3.51219805506247 3.51751682512439 3.52259342518673 3.52865552184197 3.53316807350089 3.53768062515982 3.54219317681874 3.54670572847766 3.55143972547218 3.55647692760588 3.56168247719111 3.56694531744751 3.57220815770393 3.57747099796033 3.58273383821674 3.5875530992875 3.59176313859395 3.59524803726717 3.59891401218516 3.60257998710315 3.60624596202113 3.61006223866338 3.61403025053352 3.61799826240367 3.62196627427381 3.62727855718798 3.6319884367608 3.63698876786423 3.64203407138805 3.64707937491187 3.65212467843569 3.65716998195951 3.66221528548332 3.66729939294707 3.67295160796092 3.67881814753232 3.68468468710373 3.69055122667513 3.69641776624653 3.70184846811763 3.70677938326847 3.71171029841932 3.71666876915231 3.72316392974375 3.7304733189824 3.73778270822105 3.745036871918 3.75209516011368 3.75915344830935 3.76621173650503 3.77398066542743 3.78333553443086 3.7926451126744 3.80054605529622 3.80844699791802 3.81634794053984 3.82429836269964 3.83446027504896 3.84531418436014 3.85639886265616 3.86778116509702 3.87916346753789 3.89054576997875 3.90044812182432 3.91099190865954 3.92153569549475 3.93213383878664 3.94271770825583 3.95339662764836 3.96407554704089 3.97475446643342 3.9856014296663 3.99763743545176 4.00976952670118 4.02190161795059 4.03372971668446 4.04698942952056 4.06070820502709 4.07426940349866 4.08362358507044 4.0946516607131 4.10632109738002 4.11746763572909 4.13600949794925 4.11358192572688] V  R0_mat=[0.0164025520353838,0.00991391593917779,0.00933168437168862;0.0119600956597842,0.00875043635238341,0.00956154423893035;0.0119853068610826,0.00832297953681552,0.00854455182155223;0.0111330643324705,0.00872061850253288,0.00956139374993682;0.0118222895857250,0.00795909444960185,0.00880754790179610;0.0116748342939053,0.00856548056926203,0.00938193010301517;0.0112768580015193,0.00843330788647423,0.00996649091964517;0.0118933795996695,0.00850334186162495,0.00960019659194077;0.0120321348242062,0.00846602435735512,0.00963753251603531;0.0124098156482057,0.00846539753229566,0.00929821710866923] Ohm  R0_vec=[0.056515741669998 0.0979844967251839 0.0915569898783186 0.0798231515434287 0.0702524951827934 0.0654000373090211 0.063093856936673 0.0616308263389111 0.0599710561216984 0.057768198464152 0.0561995978201733 0.0555761442485201 0.0546523884163435 0.0536806499662514 0.0531134700580429 0.0526283079740431 0.0521431458900432 0.0516579838060416 0.0515369348195236 0.0512705771965729 0.0510042195736231 0.0507378619506724 0.0504715043277217 0.0502823950776516 0.0502561644624615 0.0502595683975375 0.0502729648915397 0.0502863613855435 0.0502997578795457 0.0503131543735487 0.0503265508675508 0.0502574673059781 0.0501120429454529 0.0500297847168234 0.0499475264881939 0.0498652682595635 0.0497830100309331 0.0497007518023036 0.0496184935736741 0.0495362353450446 0.0496803807796349 0.0495816760338741 0.0494829712881124 0.0493842665423516 0.0492855617965899 0.04918685705083 0.0490881523050684 0.0489894475593067 0.0488907428135468 0.0488792431935741 0.0489051257638717 0.0489310083341703 0.0489568909044689 0.0489827734747674 0.048856619637978 0.0485561215964543 0.0482556235549287 0.0479551255134041 0.0478887983616394 0.047964487834391 0.0480401773071417 0.0480966020560407 0.0480846981417065 0.0480727942273722 0.048060890313038 0.0481036878566563 0.04837530229414 0.0486311176293377 0.0483955484453293 0.0481599792613174 0.0479244100773082 0.0476974710452733 0.0478971482990236 0.0483382198417974 0.0487792913845713 0.0492203629273451 0.0496614344701189 0.0501025060128928 0.0499772096727922 0.0499177661458976 0.049858322619003 0.0497988790921067 0.0497828516280938 0.0498086176006431 0.0498343835731925 0.0498601495457418 0.0499152254904454 0.0500578808408836 0.0502005361913236 0.0503431915417627 0.0503798029914302 0.0505673178409918 0.0508126169361116 0.0509278793074452 0.049575577643969 0.0485152342486694 0.0475667561482966 0.0457576853133315 0.0447350638775861 0.0121745905370672] Ohm  R0_dis_mat=[0.03 0.015 0.002;0.04 0.017 0.008;0.039 0.012 0.006;0.027 0.013 0.021] % Parameter not set Ohm  R0_dis_vec=[0.015 0.017 0.012 0.013] % Parameter not set Ohm  R0_ch_mat=[0.03 0.015 0.002;0.04 0.017 0.008;0.039 0.012 0.006;0.027 0.013 0.021] % Parameter not set Ohm  R0_ch_vec=[0.015 0.017 0.012 0.013] % Parameter not set Ohm  AH_vec=[1.82394991873531 2.0165 2.32772554803559] hr*A  AH=2.05260817612401 hr*A  prm_leak=ee.enum.battery.prm_leak.disabled  Rleak_vec=[8000 7000 6000] % Parameter not set Ohm  Rleak=7000 % Parameter not set Ohm  extrapolation_option=ee.enum.extrapolation.linear  prm_dyn=ee.enum.battery.prm_dyn.rc3  R1_mat=[0.00470517937000299,0.000293638394729167,0.000948546678306262;0.00290275050725254,0.000906415294998030,0.000287127543931831;0.00173884757466172,0.00126508138885500,0.00118355047696410;0.00166867739185738,0.000314621823867429,0.000269194023197089;0.000922417169458259,0.00115254740207724,0.000615957962246520;0.00120601315196432,0.000484496431848577,0.000263719105084760;0.00134107014418335,0.000722662778209487,4.84440937939109e-05;0.00102728323615524,0.000788593565891369,0.000287482375984320;0.00107112644740310,0.000808964645885711,0.000207425991333054;0.00109762911159868,0.000794632163172680,0.000106864004690497] Ohm  R1_vec=[0.076 0.022 0.007 0.043] % Parameter not set Ohm  tau1_mat=[13.5871605581300,9.71544043458337,4.31542721208131;12.5481735435305,12.1200192117783,22.7640233955017;7.48337010487386,12.0370710856561,8.29042934523224;9.44542449719648,10.9054745144726,9.51113592097300;9.24780665009956,9.25131458132309,4.68694878468948;13.0193706450093,13.4646058128269,7.73065506391290;11.2694049052077,10.2523357120003,10.8430353394808;10.5849479160592,10.0421839086956,10.9678971839482;9.25375749656255,9.65077226703459,11.6975516144793;10.0189550950196,10.0848834113777,9.87774425333310] s  tau1_vec=[148 110 27 22] % Parameter not set s  R2_mat=[0.000684064694305059,0.000979420886572540,0.000510171787438108;0.00251991269966880,0.000998429425096649,0.000143514073100964;0.00146068562126075,0.00101421826179247,0.000570655533199722;0.00169830619514015,0.00108683386499324,0.000208423134005952;0.00167031143922319,0.000980618529905995,0.000651263003556613;0.000940978707058922,0.000878005470765354,0.000327115321338108;0.000987171552806869,0.000893842003198636,9.25394354022508e-05;0.00105023394930685,0.000992613735542309,0.000107350277866256;0.00104040490708932,0.000868081363505911,9.60282071092013e-05;0.000906032230510198,0.000913369768442737,0.000476753719169488] Ohm  R2_vec=[0.382 0.006 0.007 0.956] % Parameter not set Ohm  tau2_mat=[50.0886429204366,61.4453898981661,145.884876037851;74.6890198323087,50.4659345461731,86.1376304381821;97.3437456249129,84.5850607625997,46.7659950347051;69.5883917264204,54.8647909590588,95.8259882470036;84.2274457727954,55.6603698124908,49.8887181712856;85.6679398764468,66.7955372911173,100.658737711864;91.0542017364846,92.0037411543702,98.7286168651434;105.401951521745,81.0404007236597,142.459568124630;96.5977974872106,90.8335209230926,115.401022170525;93.3993331962355,104.582879809587,83.7886054703847] s  tau2_vec=[44 24 14 13419] % Parameter not set s  R3_mat=[0.00647728107284730,0.00265301875816448,0.00382437341121983;0.00361737977004768,0.00111981676039765,0.00335084458017034;0.00344585619669106,0.00161752813625906,6.99540921903032e-05;0.00315346597824661,0.00130153280759591,0.00128660807490130;0.00209410692411210,0.00175471389437080,0.000316666511381357;0.00191509386455154,0.000370366587789619,0.000335793536625847;0.000572834619148222,0.000925138687019395,0.000330091526981303;0.00113886835462710,0.000867792101494099,0.000801284291305556;0.00101072488301601,0.000662353437832612,1.76827486513599e-05;0.00109338554767636,0.000329888238858683,7.93589066577793e-05] Ohm  R3_vec=[0.382 0.006 0.007 0.956] % Parameter not set Ohm  tau3_mat=[701.994643225609,650.007334256828,4085.79825438844;925.823429071832,649.854940905500,4973.41475833222;789.333229923387,938.725273795671,279.002198521502;654.594564127694,349.419044951255,894.440824445244;541.309382097595,983.444269794273,2138.18581380245;689.289031846017,958.570032564448,882.678111947643;601.673035616931,962.088556655044,358.867760831677;466.377911573388,402.220930598748,253.373956799259;329.012511634609,405.712600993442,527.026256725996;499.960911848800,568.259886582724,628.422969338960] s  tau3_vec=[44 24 14 13419] % Parameter not set s  R4_mat=[0.014 0.382 0.407;0.028 0.006 0.007;0.014 0.007 0.006;0.333 0.956 0.912] % Parameter not set Ohm  R4_vec=[0.382 0.006 0.007 0.956] % Parameter not set Ohm  tau4_mat=[1 44 5644;11 24 506;2 14 330;3310 13419 30216] % Parameter not set s  tau4_vec=[44 24 14 13419] % Parameter not set s  R5_mat=[0.014 0.382 0.407;0.028 0.006 0.007;0.014 0.007 0.006;0.333 0.956 0.912] % Parameter not set Ohm  R5_vec=[0.382 0.006 0.007 0.956] % Parameter not set Ohm  tau5_mat=[1 44 5644;11 24 506;2 14 330;3310 13419 30216] % Parameter not set s  tau5_vec=[44 24 14 13419] % Parameter not set s  prm_fade=ee.enum.battery.prm_fade.equations  N0=100 % Parameter not set  dV0=0 % Parameter not set  dR0=0 % Parameter not set  dAH=0 % Parameter not set  dRleak=0 % Parameter not set  dR1=0 % Parameter not set  dR2=0 % Parameter not set  dR3=0 % Parameter not set  dR4=0 % Parameter not set  dR5=0 % Parameter not set  N0vec=[1 7 13 19 25 31 37 43 49 55 61 67 73 79 85 91 97 103 109 115 121 127 133 139 145 151 157 163 169 175 181 187 193 199 205 211 217 223 229 235 241 247 253 259 265 271 277 283 289 295 301 307 313 319 325 331 337 343 349 355 361 367 373 379 385 391 397 403 409 415 421 427 433 439 445 451 457 463 469 475 481 487 493 499]  Tfadevec=[298.15 323.15] % Parameter not set K  dV0vec=[0 0.11971976024812 0.239439520496219 0.359159280744318 0.478879040992438 0.501067226691431 0.402089625480699 0.303112024269989 0.204134423059257 0.107430319615636 0.0613178904713528 0.0203784059293676 -0.0205610786126608 -0.061500563154646 -0.102440047696653 -0.14337953223866 -0.201539559021902 -0.314370645177291 -0.4272017313327 -0.535644559188378 -0.642274363906691 -0.745773535175882 -0.83621855809896 -0.926663581022039 -1.04473766830393 -1.17586008635983 -1.2842177466678 -1.38421479409414 -1.48422494017385 -1.58423508625356 -1.68205677034908 -1.77872034043833 -1.87538391052757 -1.96871527598932 -2.05494235082241 -2.14116942565553 -2.22342333172441 -2.30746775676303 -2.3916483637309 -2.47582897069879 -2.56000957766668 -2.64419018463457 -2.72837079160248 -2.81255139857038 -2.89611302552253 -2.97962692693163 -3.06874730213896 -3.15533627389878 -3.23773436162621 -3.32013244935364 -3.4021017936101 -3.48322334975892 -3.56434490590772 -3.64546646205654 -3.72658801820533 -3.8077095743541 -3.86254494056368 -3.91405004441099 -3.96555514825832 -4.01706025210565 -4.06856535595298 -4.1200704598003 -4.17141610474255 -4.23129042669511 -4.30051147066416 -4.36973251463322 -4.43899132382803 -4.50830572201986 -4.57762012021168 -4.64693451840349 -4.7160044748888 -4.7804348165123 -4.8441936541821 -4.9079524918519 -4.97171132952168 -5.03547016719147 -5.09922900486127 -5.16844365985214 -5.2420874206298 -5.31495381814591 -5.38782021566204 -5.46647669730484 -5.55023330252746 -5.63398990775009]  dR0vec=[0;0;0;0;0;0;0;0;0;0;0;0;0;0;0;0;0;0;0;0;0;0;0;0;0;0;0;0;0;0;0;0;0;0;0;0;0;0;0;0;0;0;0;0;0;0;0;0;0;0;0;0;0;0;0;0;0;0;0;0;0;0;0;0;0;0;0;0;0;0;0;0;0;0;0;0;0;0;0;0;0;0;0;0] % Parameter not set  dAHvec=[0 -0.219585533835757 -0.439171067671514 -0.658756601507271 -0.878342135343028 -1.09792766917876 -1.31751320301452 -1.53709873685028 -1.75668427068601 -1.97122596415023 -2.1223113669781 -2.27339676980596 -2.42448217263385 -2.57556757546173 -2.7266529782896 -2.87773838111746 -3.08823618102998 -3.48597596052145 -3.88371574001296 -4.28145551950445 -4.67919529899595 -5.07693507848744 -5.47467485797895 -5.87241463747045 -6.27015441696194 -6.66789419645344 -6.9965805687467 -7.29646150863608 -7.59634244852543 -7.89622338841479 -8.19610432830414 -8.49598526819352 -8.79586620808287 -9.09574714797224 -9.3956280878616 -9.69550902775097 -9.98157206200379 -10.2670000366216 -10.5524280112395 -10.8378559858573 -11.1232839604752 -11.408711935093 -11.6941399097109 -11.9795678843287 -12.2649958589466 -12.5504238335644 -12.8550132224376 -13.1674981798519 -13.4799831372661 -13.7924680946804 -14.1049530520947 -14.417438009509 -14.7299229669232 -15.0424079243375 -15.3548928817518 -15.6673778391661 -15.8786068624772 -16.0770075212716 -16.275408180066 -16.4738088388604 -16.6722094976548 -16.8706101564492 -17.0690108152436 -17.3017214786887 -17.5707595995574 -17.8397977204261 -18.1088358412948 -18.3778739621634 -18.6469120830321 -18.9159502039008 -19.1849883247695 -19.4363586274065 -19.6851091060939 -19.9338595847813 -20.1826100634686 -20.431360542156 -20.6801110208434 -20.9501469749229 -21.252844657746 -21.5555423405691 -21.8582400233922 -22.1609377062153 -22.4636353890384 -22.7663330718615]  dRleakvec=[0 0 0] % Parameter not set  dR1vec=[0 0 0] % Parameter not set  dR2vec=[0 0 0] % Parameter not set  dR3vec=[0 0 0] % Parameter not set  dR4vec=[0 0 0] % Parameter not set  dR5vec=[0 0 0] % Parameter not set  dV0mat=[0 0;0 0;0 0] % Parameter not set  dR0mat=[0 0;0 0;0 0] % Parameter not set  dAHmat=[0 0;0 0;0 0] % Parameter not set  dRleakmat=[0 0;0 0;0 0] % Parameter not set  dR1mat=[0 0;0 0;0 0] % Parameter not set  dR2mat=[0 0;0 0;0 0] % Parameter not set  dR3mat=[0 0;0 0;0 0] % Parameter not set  dR4mat=[0 0;0 0;0 0] % Parameter not set  dR5mat=[0 0;0 0;0 0] % Parameter not set  temperature=298.15 K  i_specify=off  i_priority=None  i=0 A  i_nominal_specify=off  i_nominal_unit=A  i_nominal_value=1  v_specify=off  v_priority=None  v=0 V  v_nominal_specify=off  v_nominal_unit=V  v_nominal_value=1  stateOfCharge_specify=on  stateOfCharge_priority=High  stateOfCharge=0.5  stateOfCharge_nominal_specify=off  stateOfCharge_nominal_unit=1  stateOfCharge_nominal_value=1  num_cycles_specify=off  num_cycles_priority=High  num_cycles=0  num_cycles_nominal_specify=off  num_cycles_nominal_unit=1  num_cycles_nominal_value=1  thermal_mass=30000 J/K  temperature_specify=off  temperature_priority=High  temperature_nominal_specify=off  temperature_nominal_unit=K  temperature_nominal_value=1
      settings: AttributesFormatString=UR18650A  SourceProductBaseCode=PS  InternalSimscapePortConfiguration="{\"Bottom\":[],\"Left\":[{\"id\":\"p\",\"label\":\"+\",\"type\":\"foundation.electrical.electrical\"},{\"id\":\"soc\",\"label\":\"SOC\",\"type\":\"output\"}],\"Right\":[{\"id\":\"n\",\"label\":\"-\",\"type\":\"foundation.electrical.electrical\"}],\"Top\":[]}"
  CCCV / Discharge : Subsystem
  Current Sensor : fl_lib/Electrical/Electrical Sensors/Current Sensor
  Current Sensor1 : fl_lib/Electrical/Electrical Sensors/Current Sensor
  Current Sensor2 : fl_lib/Electrical/Electrical Sensors/Current Sensor
  D1 : fl_lib/Electrical/Electrical Elements/Diode  Vf=0.6 V  Ron=0.3 Ohm  Goff=1e-8 1/Ohm  i_specify=off  i_priority=None  i=0 A  i_nominal_specify=off  i_nominal_unit=A  i_nominal_value=1  v_specify=off  v_priority=None  v=0 V  v_nominal_specify=off  v_nominal_unit=V  v_nominal_value=1
      settings: LogSimulationData=on
  D2 : fl_lib/Electrical/Electrical Elements/Diode  Vf=0.6 V  Ron=0.3 Ohm  Goff=1e-8 1/Ohm  i_specify=off  i_priority=None  i=0 A  i_nominal_specify=off  i_nominal_unit=A  i_nominal_value=1  v_specify=off  v_priority=None  v=0 V  v_nominal_specify=off  v_nominal_unit=V  v_nominal_value=1
      settings: LogSimulationData=on
  D3 : fl_lib/Electrical/Electrical Elements/Diode  Vf=0.6 V  Ron=0.3 Ohm  Goff=1e-8 1/Ohm  i_specify=off  i_priority=None  i=0 A  i_nominal_specify=off  i_nominal_unit=A  i_nominal_value=1  v_specify=off  v_priority=None  v=0 V  v_nominal_specify=off  v_nominal_unit=V  v_nominal_value=1
      settings: LogSimulationData=on
  Electrical Reference : fl_lib/Electrical/Electrical Elements/Electrical Reference
  FET1 : ee_lib/Semiconductors & Converters/MOSFET (Ideal, Switching)  Rds=0.01 Ohm  Goff=1e-6 1/Ohm  Vth=0.9 V  diode_param=2  diode_Vf=0.8 V  diode_Ron=0.001 Ohm  diode_Goff=1e-5 1/Ohm  diode_C=5e-8 F  diode_iRM=-235 A  diode_iF=300 A  diode_idot=-50 A/us  diode_trr_param=1  diode_trr_factor=3  diode_trr=15 us  diode_Qrr=1.5e+3 s*uA  thermal_loss_option=2  Von_data=[0, 1.1, 1.3, 1.45, 1.75, 2.25, 2.7; 0, 1, 1.15, 1.35, 1.7, 2.35, 3] V  Eon_data=[0, .29, 1.43, 2.86, 5.71, 13.14, 22.86; 0, .57, 2.63, 5.14, 10.29, 20.57, 30.29] * 1e-3 J  Eoff_data=[0, .21, 1.07, 2.14, 4.29, 9.86, 17.14; 0, .43, 1.97, 3.86, 7.71, 15.43, 22.71] * 1e-3 J  Tj=[298.15, 398.15] K  Iout_data=[0, 10, 50, 100, 200, 400, 600] A  Eon_scalar=22.86e-3 J  Eoff_scalar=17.14e-3 J  Voff=300 V  Iout_scalar=600 A  diodeModelType=ee.enum.converters.diodeModelType.pwl  diode_IfMat=[.07, .12, .19, 1.75, 4.24, 7.32, 11.2; .16, .3, .72, 2.14, 4.02, 6.35, 9.12] A  diode_TjVec=[25, 125] degC  diode_VfVec=[.5, .7, .9, 1.3, 1.7, 2.1, 2.5] V  thermal_network_parameterization=ee.enum.thermalNetworkTopology.external  Rth=[.03, .2] K/W  Rth_Foster=[.03, .2] K/W  thermal_mass_parameterization=ee.enum.thermalNetwork.timeconstant  thermal_mass=[3, 25] J/K  thermal_mass_Foster=[33, 50] J/K  thermal_time_constant=[.1, 5] s  thermal_time_constant_Foster=[1, 10] s  thermal_mass_initial_temperatures=[25, 25] degC  junction_thermal_mass=0.1 J/K  Tau=1e-4 s  vT_specify=off  vT_priority=None  vT=0 V  vT_nominal_specify=off  vT_nominal_unit=V  vT_nominal_value=1  Qj_specify=off  Qj_priority=None  Qj=0 W  Qj_nominal_specify=off  Qj_nominal_unit=W  Qj_nominal_value=1  junction_temperature_specify=off  junction_temperature_priority=None  junction_temperature=25 degC  junction_temperature_nominal_specify=off  junction_temperature_nominal_unit=degC  junction_temperature_nominal_value=1
  FET2 : ee_lib/Semiconductors & Converters/MOSFET (Ideal, Switching)  Rds=0.01 Ohm  Goff=1e-6 1/Ohm  Vth=0.9 V  diode_param=2  diode_Vf=0.8 V  diode_Ron=0.001 Ohm  diode_Goff=1e-5 1/Ohm  diode_C=5e-8 F  diode_iRM=-235 A  diode_iF=300 A  diode_idot=-50 A/us  diode_trr_param=1  diode_trr_factor=3  diode_trr=15 us  diode_Qrr=1.5e+3 s*uA  thermal_loss_option=2  Von_data=[0, 1.1, 1.3, 1.45, 1.75, 2.25, 2.7; 0, 1, 1.15, 1.35, 1.7, 2.35, 3] V  Eon_data=[0, .29, 1.43, 2.86, 5.71, 13.14, 22.86; 0, .57, 2.63, 5.14, 10.29, 20.57, 30.29] * 1e-3 J  Eoff_data=[0, .21, 1.07, 2.14, 4.29, 9.86, 17.14; 0, .43, 1.97, 3.86, 7.71, 15.43, 22.71] * 1e-3 J  Tj=[298.15, 398.15] K  Iout_data=[0, 10, 50, 100, 200, 400, 600] A  Eon_scalar=22.86e-3 J  Eoff_scalar=17.14e-3 J  Voff=300 V  Iout_scalar=600 A  diodeModelType=ee.enum.converters.diodeModelType.pwl  diode_IfMat=[.07, .12, .19, 1.75, 4.24, 7.32, 11.2; .16, .3, .72, 2.14, 4.02, 6.35, 9.12] A  diode_TjVec=[25, 125] degC  diode_VfVec=[.5, .7, .9, 1.3, 1.7, 2.1, 2.5] V  thermal_network_parameterization=ee.enum.thermalNetworkTopology.external  Rth=[.03, .2] K/W  Rth_Foster=[.03, .2] K/W  thermal_mass_parameterization=ee.enum.thermalNetwork.timeconstant  thermal_mass=[3, 25] J/K  thermal_mass_Foster=[33, 50] J/K  thermal_time_constant=[.1, 5] s  thermal_time_constant_Foster=[1, 10] s  thermal_mass_initial_temperatures=[25, 25] degC  junction_thermal_mass=0.1 J/K  Tau=1e-4 s  vT_specify=off  vT_priority=None  vT=0 V  vT_nominal_specify=off  vT_nominal_unit=V  vT_nominal_value=1  Qj_specify=off  Qj_priority=None  Qj=0 W  Qj_nominal_specify=off  Qj_nominal_unit=W  Qj_nominal_value=1  junction_temperature_specify=off  junction_temperature_priority=None  junction_temperature=25 degC  junction_temperature_nominal_specify=off  junction_temperature_nominal_unit=degC  junction_temperature_nominal_value=1
  FET3 : ee_lib/Semiconductors & Converters/MOSFET (Ideal, Switching)  Rds=0.01 Ohm  Goff=1e-6 1/Ohm  Vth=0.9 V  diode_param=2  diode_Vf=0.8 V  diode_Ron=0.001 Ohm  diode_Goff=1e-5 1/Ohm  diode_C=5e-8 F  diode_iRM=-235 A  diode_iF=300 A  diode_idot=-50 A/us  diode_trr_param=1  diode_trr_factor=3  diode_trr=15 us  diode_Qrr=1.5e+3 s*uA  thermal_loss_option=2  Von_data=[0, 1.1, 1.3, 1.45, 1.75, 2.25, 2.7; 0, 1, 1.15, 1.35, 1.7, 2.35, 3] V  Eon_data=[0, .29, 1.43, 2.86, 5.71, 13.14, 22.86; 0, .57, 2.63, 5.14, 10.29, 20.57, 30.29] * 1e-3 J  Eoff_data=[0, .21, 1.07, 2.14, 4.29, 9.86, 17.14; 0, .43, 1.97, 3.86, 7.71, 15.43, 22.71] * 1e-3 J  Tj=[298.15, 398.15] K  Iout_data=[0, 10, 50, 100, 200, 400, 600] A  Eon_scalar=22.86e-3 J  Eoff_scalar=17.14e-3 J  Voff=300 V  Iout_scalar=600 A  diodeModelType=ee.enum.converters.diodeModelType.pwl  diode_IfMat=[.07, .12, .19, 1.75, 4.24, 7.32, 11.2; .16, .3, .72, 2.14, 4.02, 6.35, 9.12] A  diode_TjVec=[25, 125] degC  diode_VfVec=[.5, .7, .9, 1.3, 1.7, 2.1, 2.5] V  thermal_network_parameterization=ee.enum.thermalNetworkTopology.external  Rth=[.03, .2] K/W  Rth_Foster=[.03, .2] K/W  thermal_mass_parameterization=ee.enum.thermalNetwork.timeconstant  thermal_mass=[3, 25] J/K  thermal_mass_Foster=[33, 50] J/K  thermal_time_constant=[.1, 5] s  thermal_time_constant_Foster=[1, 10] s  thermal_mass_initial_temperatures=[25, 25] degC  junction_thermal_mass=0.1 J/K  Tau=1e-4 s  vT_specify=off  vT_priority=None  vT=0 V  vT_nominal_specify=off  vT_nominal_unit=V  vT_nominal_value=1  Qj_specify=off  Qj_priority=None  Qj=0 W  Qj_nominal_specify=off  Qj_nominal_unit=W  Qj_nominal_value=1  junction_temperature_specify=off  junction_temperature_priority=None  junction_temperature=25 degC  junction_temperature_nominal_specify=off  junction_temperature_nominal_unit=degC  junction_temperature_nominal_value=1
  I_TOT : fl_lib/Electrical/Electrical Sources/Controlled Current Source
  PS-Simulink Converter{1..8,10,13} (10 alike) : nesl_utility/PS-Simulink Converter  PhysicalDomain=network_engine_domain  SubClassName=ps_output  LeftPortType=input  RightPortType=output  PseudoPeriodic=off  Frequencies=[]  Unit=1  AffineConversion=off
  R1 : fl_lib/Electrical/Electrical Elements/Resistor  R=R_bleed Ohm  i_specify=off  i_priority=None  i=0 A  i_nominal_specify=off  i_nominal_unit=A  i_nominal_value=1  v_specify=off  v_priority=None  v=0 V  v_nominal_specify=off  v_nominal_unit=V  v_nominal_value=1
      settings: LogSimulationData=on
  R2 : fl_lib/Electrical/Electrical Elements/Resistor  R=R_bleed Ohm  i_specify=off  i_priority=None  i=0 A  i_nominal_specify=off  i_nominal_unit=A  i_nominal_value=1  v_specify=off  v_priority=None  v=0 V  v_nominal_specify=off  v_nominal_unit=V  v_nominal_value=1
  R3 : fl_lib/Electrical/Electrical Elements/Resistor  R=R_bleed Ohm  i_specify=off  i_priority=None  i=0 A  i_nominal_specify=off  i_nominal_unit=A  i_nominal_value=1  v_specify=off  v_priority=None  v=0 V  v_nominal_specify=off  v_nominal_unit=V  v_nominal_value=1
  Scopes : Subsystem
  Simulink-PS Converter : nesl_utility/Simulink-PS Converter  PhysicalDomain=network_engine_domain  SubClassName=ps_input  LeftPortType=input  RightPortType=output  PseudoPeriodic=off  Frequencies=[]  NoiseDistribution=none  NoiseParameters=[]  Unit=1  AffineConversion=off  FilteringAndDerivatives=provide  SimscapeFilterOrder=1  InputFilterTimeConstant=0.001  UdotUserProvided=0
  Simulink-PS Converter1 : nesl_utility/Simulink-PS Converter  PhysicalDomain=network_engine_domain  SubClassName=ps_input  LeftPortType=input  RightPortType=output  PseudoPeriodic=off  Frequencies=[]  NoiseDistribution=none  NoiseParameters=[]  Unit=1  AffineConversion=off  FilteringAndDerivatives=zero  SimscapeFilterOrder=1  InputFilterTimeConstant=0.001  UdotUserProvided=1
  Simulink-PS Converter2 : nesl_utility/Simulink-PS Converter  PhysicalDomain=network_engine_domain  SubClassName=ps_input  LeftPortType=input  RightPortType=output  PseudoPeriodic=off  Frequencies=[]  NoiseDistribution=none  NoiseParameters=[]  Unit=1  AffineConversion=off  FilteringAndDerivatives=zero  SimscapeFilterOrder=1  InputFilterTimeConstant=0.001  UdotUserProvided=1
  Simulink-PS Converter3 : nesl_utility/Simulink-PS Converter  PhysicalDomain=network_engine_domain  SubClassName=ps_input  LeftPortType=input  RightPortType=output  PseudoPeriodic=off  Frequencies=[]  NoiseDistribution=none  NoiseParameters=[]  Unit=1  AffineConversion=off  FilteringAndDerivatives=zero  SimscapeFilterOrder=1  InputFilterTimeConstant=0.001  UdotUserProvided=1
  Solver Configuration : nesl_utility/Solver Configuration  PhysicalDomain=network_engine_domain  SubClassName=solver  LeftPortType=input  RightPortType=generic  Tones=[]  Harmonics=[]  SimulateNoise=off  Profile=off  UseLocalSampling=off  EnableSwitchedLinearOptims=on  FrequencyDomain=off  UseCCode=off  RelTol=0.001  AbsTol=1e-06  MinStep=1e-09  ToWorkspace=off  RevertToSquareIcSolve=off  NumHomotopyIterations=100  PhasorMode=off  PhasorModeNumHarmonics=1  DoDC=off  ResidualTolerance=1e-09  UseLocalSolver=on  LocalSolverChoice=NE_BACKWARD_EULER_ADVANCER  LocalSolverSampleTime=1  DoFixedCost=on  MaxNonlinIter=3  MaxModeIter=2  ComputeImpulses=off  ImpulseIterations=2  LinearAlgebra=Sparse  EquationFormulation=NE_TIME_EF  DelaysMemoryBudget=1024  AutomaticFiltering=on  FilteringTimeConstant=0.001  PartitionStorageMethod=AS_NEEDED  PartitionMemoryBudget=1024  PartitionMethod=FAST
  Transfer Fcn1 : TransferFcn  Denominator=[T_f 1]
  Transfer Fcn2 : TransferFcn  Denominator=[T_f 1]
  Transfer Fcn3 : TransferFcn  Denominator=[T_f 1]
  Voltage Sensor{1..4} (4 alike) : fl_lib/Electrical/Electrical Sensors/Voltage Sensor
  balancing logic : Stateflow chart  TreatAsAtomicUnit=on  VariantControl=(default)
  tag scope: I1=global, I2=global, I3=global, I=global, SOC_1=global, SOC_2=global, SOC_3=global, V1=global, V2=global, V3=global, V=global
  wires:
  PS-Simulink Converter6/1 -> [SOC_2]
  balancing logic/3(s3) -> Simulink-PS Converter3/1
  PS-Simulink Converter7/1 -> [SOC_3]
  Transfer Fcn3/1 -> balancing logic/3(v3)
  PS-Simulink Converter3/1 -> [V1]
  PS-Simulink Converter5/1 -> [SOC_1]
  [V2] -> Transfer Fcn1/1
  [V3] -> Transfer Fcn3/1
  Transfer Fcn1/1 -> balancing logic/2(v2)
  balancing logic/1(s1) -> Simulink-PS Converter2/1
  balancing logic/2(s2) -> Simulink-PS Converter1/1
  PS-Simulink Converter8/1 -> [I1]
  PS-Simulink Converter2/1 -> [V]
  [V1] -> Transfer Fcn2/1
  Transfer Fcn2/1 -> balancing logic/1(v1)
  PS-Simulink Converter1/1 -> [V2]
  PS-Simulink Converter10/1 -> [I2]
  PS-Simulink Converter4/1 -> [V3]
  PS-Simulink Converter13/1 -> [I3]
  CCCV / Discharge/1(Out1) -> Simulink-PS Converter/1, [I]
  connections:
  Voltage Sensor1/RConn1 -- PS-Simulink Converter2/LConn1
  Simulink-PS Converter/RConn1 -- I_TOT/RConn1
  Current Sensor1/LConn1 -- Battery (Table-Based)1/RConn1 -- R2/LConn1 -- FET1/RConn2 -- Voltage Sensor3/LConn1 -- Voltage Sensor2/RConn2
  Battery (Table-Based)2/RConn1 -- Current Sensor2/LConn1 -- Voltage Sensor4/LConn1 -- Voltage Sensor3/RConn2 -- R3/LConn1 -- FET2/RConn2
  I_TOT/RConn2 -- Voltage Sensor4/RConn2 -- FET3/RConn2 -- Battery (Table-Based)3/RConn1 -- Electrical Reference/LConn1 -- Solver Configuration/RConn1 -- Voltage Sensor1/RConn2
  Voltage Sensor1/LConn1 -- I_TOT/LConn1 -- R1/LConn1 -- Voltage Sensor2/LConn1 -- Current Sensor/LConn1
  R1/RConn1 -- D1/LConn1
  FET1/RConn1 -- D1/RConn1
  Battery (Table-Based)3/LConn2 -- PS-Simulink Converter7/LConn1
  Battery (Table-Based)2/LConn2 -- PS-Simulink Converter6/LConn1
  FET3/RConn1 -- D3/RConn1
  Battery (Table-Based)1/LConn2 -- PS-Simulink Converter5/LConn1
  Simulink-PS Converter3/RConn1 -- FET3/LConn1
  PS-Simulink Converter1/LConn1 -- Voltage Sensor3/RConn1
  Battery (Table-Based)3/LConn1 -- Current Sensor2/RConn2
  R3/RConn1 -- D3/LConn1
  Battery (Table-Based)1/LConn1 -- Current Sensor/RConn2
  PS-Simulink Converter4/LConn1 -- Voltage Sensor4/RConn1
  R2/RConn1 -- D2/LConn1
  PS-Simulink Converter3/LConn1 -- Voltage Sensor2/RConn1
  Simulink-PS Converter2/RConn1 -- FET1/LConn1
  Simulink-PS Converter1/RConn1 -- FET2/LConn1
  FET2/RConn1 -- D2/RConn1
  PS-Simulink Converter8/LConn1 -- Current Sensor/RConn1
  Battery (Table-Based)2/LConn1 -- Current Sensor1/RConn2
  PS-Simulink Converter10/LConn1 -- Current Sensor1/RConn1
  Current Sensor2/RConn1 -- PS-Simulink Converter13/LConn1
